simulink model "seguimiento_constante_nominal_modelo_lineal"  (R2021a)
settings: Solver=VariableStepAuto  StartTime=0.0  StopTime=15  RelTol=1e-3
settings Model: Creator=jmata  LastModifiedBy=jmata

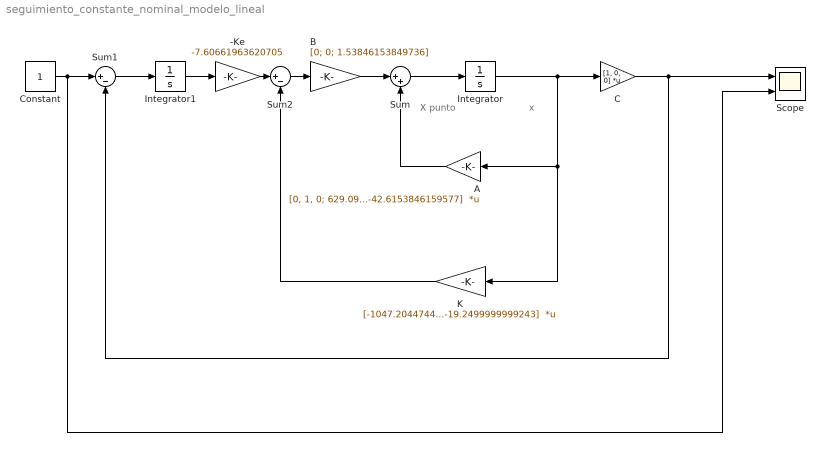
== system seguimiento_constante_nominal_modelo_lineal ==
  note: x
  note: X punto
  -Ke : Gain  Gain=-7.60661963620705
  "A " : Gain  Gain="[0, 1, 0; 629.09300494194, 0, -5.12711320724338;  0, 0, -42.6153846159577]"  Multiplication=Matrix(K*u)
  "B " : Gain  Gain=[0; 0; 1.53846153849736]
  "C " : Gain  Gain=[1, 0, 0]  Multiplication=Matrix(K*u)
  Constant : Constant
  Integrator : Integrator
  Integrator1 : Integrator
  K : Gain  Gain=[-1047.2044744495, -86.6004777453798, -19.2499999999243]  Multiplication=Matrix(K*u)
  Scope : Scope  NumInputPorts=2
  Sum : Sum  Inputs=|++
  Sum1 : Sum  Inputs=|+-
  Sum2 : Sum  Inputs=|+-
  wires:
  "B "/1 -> Sum/1
  Sum/1 -> Integrator/1
  Integrator1/1 -> -Ke/1
  Sum2/1 -> "B "/1
  Constant/1 -> Scope/2, Sum1/1
  K/1 -> Sum2/2
  Integrator/1 -> K/1, "A "/1, "C "/1
  "A "/1 -> Sum/2
  -Ke/1 -> Sum2/1
  Sum1/1 -> Integrator1/1
  "C "/1 -> Sum1/2, Scope/1
